simulink model "model_ogrzewania"  (R2018b)
settings: Solver=VariableStepAuto  StartTime=0.0  StopTime=4000  RelTol=1e-3
values from neighbouring files (symbols this model uses):
  ap = 25.96    [calculate_T.m]    (also in calculate_dpsi1.m; calculate_dpsi2.m; main.m)
  as = 6.47    [calculate_Ts.m]    (also in calculate_dpsi1.m; calculate_dpsi2.m; main.m)
  kf = 4.62    [calculate_T.m]    (also in calculate_dpsi1.m; calculate_dpsi2.m; main.m)
  taup = 53.7    [calculate_T.m]    (also in calculate_dpsi1.m; calculate_dpsi2.m; main.m)
  taus = 153.54    [calculate_Ts.m]    (also in calculate_dpsi1.m; calculate_dpsi2.m; main.m)
  time = zeros(1, length(T_zewn))    [main.m]
undefined symbols (not defined in the file or in its folder): Tref, Tzco, Tzewn
libraries: simulink x3
settings Model: Creator=aleks  LastModifiedBy=aleks

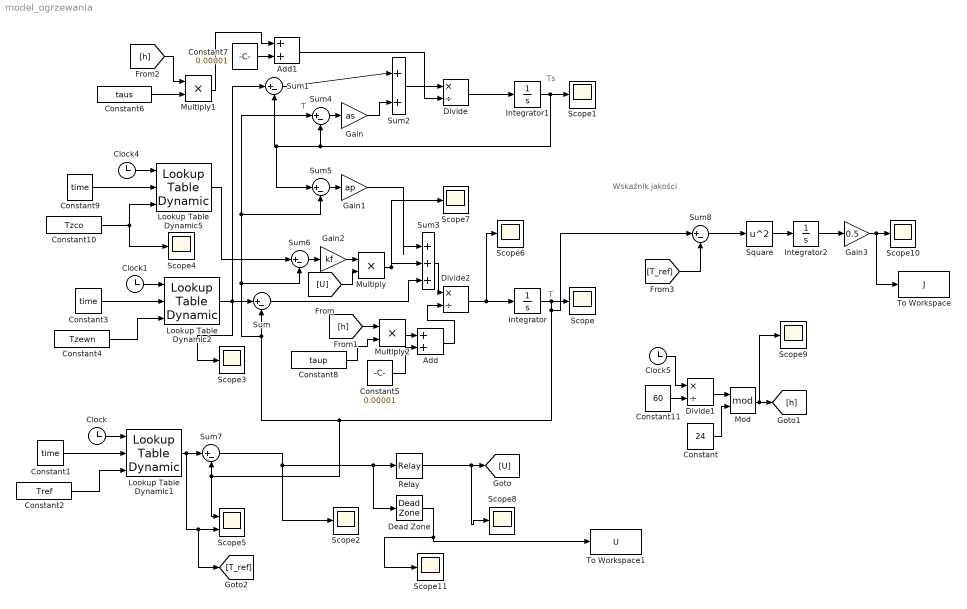
== system model_ogrzewania ==
  note: Wskaźnik jakości
  note: T
  note: T
  note: Ts
  Add : Sum
  Add1 : Sum
  Clock{,1,4..5} (4 alike) : Clock
  Constant : Constant  Value=24
  Constant1 : Constant  Value=time
  Constant10 : Constant  Value=Tzco
  Constant11 : Constant  Value=60
  Constant2 : Constant  Value=Tref
  Constant3 : Constant  Value=time
  Constant4 : Constant  Value=Tzewn
  Constant5 : Constant  Value=0.00001
  Constant6 : Constant  Value=taus
  Constant7 : Constant  Value=0.00001
  Constant8 : Constant  Value=taup
  Constant9 : Constant  Value=time
  Dead Zone : DeadZone  LowerValue=-2  UpperValue=2  SaturateOnIntegerOverflow=on
  Divide : Product  Inputs=*/
  Divide1 : Product  Inputs=*/
  Divide2 : Product  Inputs=*/
  Gain : Gain  Gain=as
  Gain1 : Gain  Gain=ap
  Gain2 : Gain  Gain=kf
  Gain3 : Gain  Gain=0.5
  Integrator : Integrator  InitialCondition=20
  Integrator1 : Integrator
  Integrator2 : Integrator
  Lookup Table Dynamic1 : simulink/Lookup Tables/Lookup Table Dynamic  LookUpMeth=Interpolation-Use End Values  OutDataType=fixdt('double')  OutScaling=[]  OutputDataTypeScalingMode=Specify via dialog  OutDataTypeStr=double  DoSatur=off
      settings: SourceProductName=Simulink
  Lookup Table Dynamic2 : simulink/Lookup Tables/Lookup Table Dynamic  LookUpMeth=Interpolation-Use End Values  OutDataType=fixdt('double')  OutScaling=[]  OutputDataTypeScalingMode=Specify via dialog  OutDataTypeStr=double  DoSatur=off
      settings: SourceProductName=Simulink
  Lookup Table Dynamic5 : simulink/Lookup Tables/Lookup Table Dynamic  LookUpMeth=Interpolation-Use End Values  OutDataType=fixdt('double')  OutScaling=[]  OutputDataTypeScalingMode=Specify via dialog  OutDataTypeStr=double  DoSatur=off
      settings: SourceProductName=Simulink
  Mod : Math  Operator=mod  SaturateOnIntegerOverflow=on
  Multiply : Product
  Multiply1 : Product
  Multiply2 : Product
  Relay : Relay  OnSwitchValue=3  OffSwitchValue=-3
  Scope{,1..4,6..11} (11 alike) : Scope
  Scope5 : Scope  NumInputPorts=2
  Square : Math  Operator=square  SaturateOnIntegerOverflow=on
  Sum{,1,4..8} (7 alike) : Sum  Inputs=|+-
  Sum2 : Sum  Inputs=|++
  Sum3 : Sum  Inputs=|+++
  To Workspace : ToWorkspace  VariableName=J  SaveFormat=Timeseries  SampleTime=-1
  To Workspace1 : ToWorkspace  VariableName=U  SaveFormat=Timeseries  SampleTime=-1
  wires:
  Constant1/1 -> Lookup Table Dynamic1/2
  Clock/1 -> Lookup Table Dynamic1/1
  Constant2/1 -> Lookup Table Dynamic1/3
  Constant3/1 -> Lookup Table Dynamic2/2
  Constant4/1 -> Lookup Table Dynamic2/3
  Clock1/1 -> Lookup Table Dynamic2/1
  Lookup Table Dynamic2/1 -> Scope3/1, Sum1/1, Sum/1
  Integrator1/1 -> Sum4/2, Sum5/1, Sum1/2, Scope1/1
  Constant6/1 -> Multiply1/2
  Sum1/1 -> Sum2/1
  Sum4/1 -> Gain/1
  Gain/1 -> Sum2/2
  Constant8/1 -> Multiply2/2
  Sum2/1 -> Divide/1
  Divide/1 -> Integrator1/1
  Sum3/1 -> Divide2/1
  Divide2/1 -> Scope6/1, Integrator/1
  Sum/1 -> Sum3/3
  Sum5/1 -> Gain1/1
  Gain1/1 -> Sum3/1
  Constant10/1 -> Lookup Table Dynamic5/3, Scope4/1
  Clock4/1 -> Lookup Table Dynamic5/1
  Constant9/1 -> Lookup Table Dynamic5/2
  Lookup Table Dynamic5/1 -> Sum6/1
  Sum6/1 -> Gain2/1
  Gain2/1 -> Multiply/1
  Multiply/1 -> Scope7/1, Sum3/2
  [U] -> Multiply/2
  Multiply2/1 -> Add/1
  Add/1 -> Divide2/2
  Constant5/1 -> Add/2
  Constant7/1 -> Add1/2
  Multiply1/1 -> Add1/1
  Add1/1 -> Divide/2
  Lookup Table Dynamic1/1 -> [T_ref], Scope5/2, Sum7/1
  Divide1/1 -> Mod/1
  Constant/1 -> Mod/2
  Constant11/1 -> Divide1/2
  Clock5/1 -> Divide1/1
  Mod/1 -> Scope9/1, [h]
  [h] -> Multiply2/1
  [h] -> Multiply1/1
  Relay/1 -> Scope8/1, [U]
  Sum7/1 -> Dead Zone/1, Relay/1, Scope2/1
  Integrator2/1 -> Gain3/1
  Square/1 -> Integrator2/1
  Sum8/1 -> Square/1
  [T_ref] -> Sum8/2
  Integrator/1 -> Scope/1, Sum8/1, Sum6/2, Sum5/2, Sum4/1, Sum/2, Scope5/1, Sum7/2
  Gain3/1 -> To Workspace/1, Scope10/1
  Dead Zone/1 -> To Workspace1/1, Scope11/1
